simulink model "Iface"  (R2018b)
settings: Solver=FixedStepDiscrete  StartTime=0.0  StopTime=10.0  RelTol=1e-3
undefined symbols (not defined in the file or in its folder): element_data
settings Model: Creator=matlab  LastModifiedBy=matlab
settings DataIOCC: SaveOutput=off  SignalLogging=off  SaveTime=off
settings OptimizationCC: DefaultParameterBehavior=Inlined  EnhancedBackFolding=on  PassReuseOutputArgsAs=Individual arguments  OptimizeBlockOrder=speed  DifferentSizesBufferReuse=on  OptimizationCustomize=off
settings DebuggingCC: ParameterTunabilityLossMsg=error
settings SFSimCC: MATLABDynamicMemAlloc=off
settings RTWCC: SystemTargetFile=ert.tlc  TemplateMakefile=ert_default_tmf  PostCodeGenCommand=packNGo(buildInfo);  GenerateReport=on  IncludeHyperlinkInReport=on  LaunchReport=on  GenerateTraceInfo=on  GenerateTraceReport=on  GenerateTraceReportSl=on  GenerateTraceReportSf=on  GenerateTraceReportEml=on
settings CodeAppCC: ForceParamTrailComments=on  IgnoreCustomStorageClasses=off  OperatorAnnotations=on  SimulinkDataObjDesc=on  SFDataObjDesc=on  InsertBlockDesc=on
settings ERTTargetCC: TargetLangStandard=C99 (ISO)  GenerateSampleERTMain=on  InlinedParameterPlacement=NonHierarchical  ERTCustomFileTemplate=example_file_process.tlc

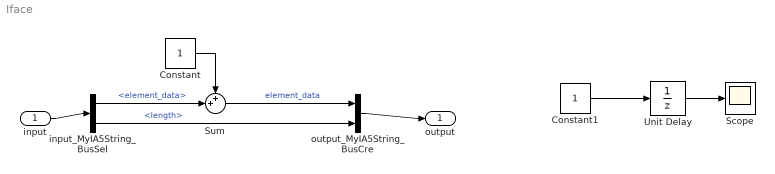
== system Iface ==
  input : Inport  OutDataTypeStr=Bus: MyIA5String  BusOutputAsStruct=on
  Constant : Constant  OutDataTypeStr=uint8
  Constant1 : Constant
  Scope : Scope
  Sum : Sum  Inputs=++|
  Unit Delay : UnitDelay  SampleTime=-1
  input_MyIA5String_BusSel : BusSelector  OutputSignals=element_data,length
  output_MyIA5String_BusCre : BusCreator  Inputs=element_data,length  OutDataTypeStr=Bus: MyIA5String  NonVirtualBus=on
  output : Outport  OutDataTypeStr=Bus: MyIA5String  BusOutputAsStruct=on
  wires:
  input/1 -> input_MyIA5String_BusSel/1
  output_MyIA5String_BusCre/1 -> output/1
  input_MyIA5String_BusSel/2 -> output_MyIA5String_BusCre/2  "<length>"
  input_MyIA5String_BusSel/1 -> Sum/2  "<element_data>"
  Sum/1 -> output_MyIA5String_BusCre/1  "element_data"
  Constant/1 -> Sum/1
  Unit Delay/1 -> Scope/1
  Constant1/1 -> Unit Delay/1
